simulink model "GearPlant"  (R2021b)
settings: Solver=VariableStepAuto  StartTime=0.0  StopTime=10.0  RelTol=1e-3
undefined symbols (not defined in the file): GearStateEnum
settings Model: Creator=david  LastModifiedBy=david

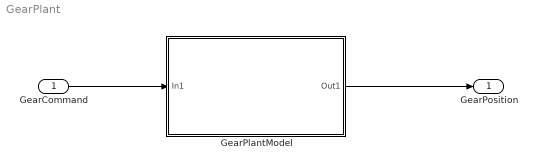
== system GearPlant ==
  GearCommand : Inport  OutDataTypeStr=Enum: GearCommandEnum
  GearPlantModel : Subsystem
  GearPosition : Outport  OutDataTypeStr=Enum: GearStateEnum
  wires:
  GearCommand/1 -> GearPlantModel/1(In1)
  GearPlantModel/1(Out1) -> GearPosition/1

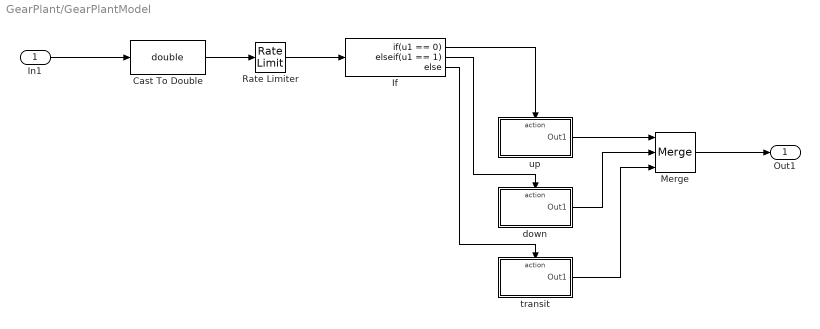
== system GearPlant/GearPlantModel ==
  In1 : Inport
  Cast To Double : DataTypeConversion  OutDataTypeStr=double
  If : If  IfExpression=u1 == 0  ElseIfExpressions=u1 == 1
  Merge : Merge  Inputs=3
  Rate Limiter : RateLimiter  RisingSlewLimit=1/5  FallingSlewLimit=-1/5
  down : Subsystem  TreatAsAtomicUnit=on
  transit : Subsystem  TreatAsAtomicUnit=on
  up : Subsystem  TreatAsAtomicUnit=on
  Out1 : Outport
  wires:
  In1/1 -> Cast To Double/1
  Cast To Double/1 -> Rate Limiter/1
  Rate Limiter/1 -> If/1
  If/1 -> up/Action
  up/1(Out1) -> Merge/1
  Merge/1 -> Out1/1
  down/1(Out1) -> Merge/2
  If/2 -> down/Action
  If/3 -> transit/Action
  transit/1(Out1) -> Merge/3

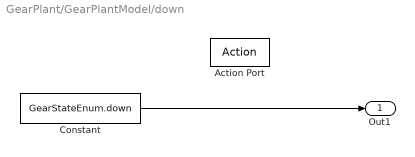
== system GearPlant/GearPlantModel/down ==
  Action Port : ActionPort  ActionPortLabel=elseif(u1 == 1)
  Constant : Constant  Value=GearStateEnum.down
  Out1 : Outport
  wires:
  Constant/1 -> Out1/1

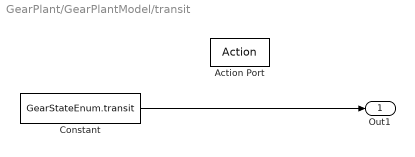
== system GearPlant/GearPlantModel/transit ==
  Action Port : ActionPort  ActionPortLabel=else
  Constant : Constant  Value=GearStateEnum.transit
  Out1 : Outport
  wires:
  Constant/1 -> Out1/1

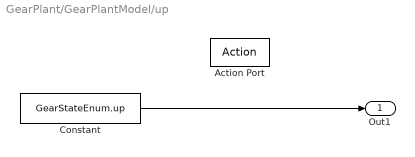
== system GearPlant/GearPlantModel/up ==
  Action Port : ActionPort  ActionPortLabel=if(u1 == 0)
  Constant : Constant  Value=GearStateEnum.up
  Out1 : Outport
  wires:
  Constant/1 -> Out1/1
